simulink model "radar_instrumentation_poc"  (R2026a)
settings: Solver=ode45  StopTime=7.67e-05  MaxStep=1e-07  RelTol=1e-5
settings Model: Creator=anamolkhadka  LastModifiedBy=anamolkhadka

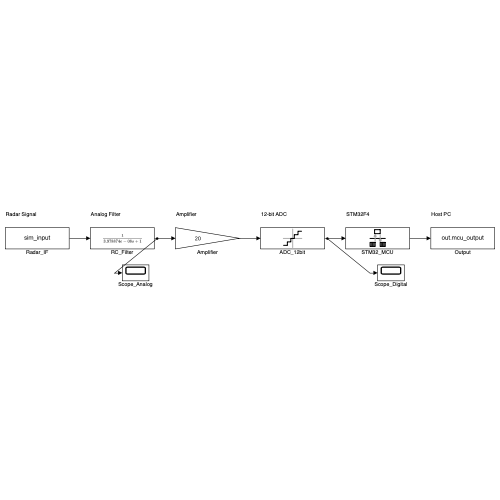
[thumbnail: Simulink's stored preview of the top-level diagram]
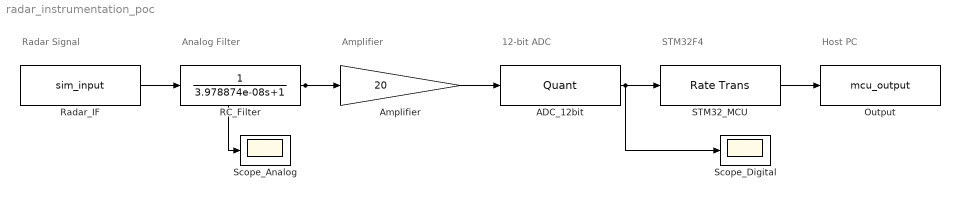
== system radar_instrumentation_poc ==
  note: Radar Signal
  note: Analog Filter
  note: Amplifier
  note: 12-bit ADC
  note: STM32F4
  note: Host PC
  ADC_12bit : Quantizer  QuantizationInterval=0.00080586
  Amplifier : Gain  Gain=20
  Output : ToWorkspace  VariableName=mcu_output  SaveFormat=Timeseries  SampleTime=-1
  RC_Filter : TransferFcn  Denominator=[3.978874e-08 1]
  Radar_IF : FromWorkspace  VariableName=sim_input  SampleTime=1e-07
  STM32_MCU : RateTransition
  Scope_Analog : Scope
  Scope_Digital : Scope
  wires:
  Radar_IF/1 -> RC_Filter/1
  RC_Filter/1 -> Amplifier/1, Scope_Analog/1
  Amplifier/1 -> ADC_12bit/1
  ADC_12bit/1 -> STM32_MCU/1, Scope_Digital/1
  STM32_MCU/1 -> Output/1
